simulink model "gimbal_model"  (R2016b)
settings: Solver=VariableStepAuto  StartTime=0.0  StopTime=60  RelTol=1e-3
values from neighbouring files (symbols this model uses):
  A = J*(Omega_phi + Omega)    [IMU.m]
  DIM = data{4}    [gimbal_dynamics.m]
  DIS = data{5}    [gimbal_dynamics.m]
  I1 = data{1}    [gimbal_dynamics.m]    (also in macierze_inercji.m = sym('I1', [4 4]))
  I2 = data{2}    [gimbal_dynamics.m]    (also in macierze_inercji.m = sym('I2', [4 4]))
  I3 = data{3}    [gimbal_dynamics.m]    (also in macierze_inercji.m = sym('I3', [4 4]))
  M = [ud_ucz(3:p-1) ud_ucz(3:p-1).^2 ud_ucz(3:p-1).^3 ud_ucz(2:p-2) ud_ucz(2:p-2).^2 ud_ucz(2:p-2).^3 ud_ucz(1:p-3) ud_ucz(1:p-3).^2 ud_ucz(1:p-3).^3 yd_ucz(3:p-1) yd_ucz(3:p-1).^2 yd_ucz(3:p-1).^3 yd_ucz(2:p-2) yd_ucz(2:p-2).^2 yd_ucz(2:p-2).^3 yd_ucz(1:p-3) yd_ucz(1:p-3).^2 yd_ucz(1:p-3).^3]    [Identification_20191023.m]    (also in MI_beta.m = fillmissing(M,'spline'); gimbal_dynamics.m = data{6}; macierze_inercji.m = sym('M', [1 3]))
  phase = 6    [calculate_PWM.m]    (also in pwm_test.m)
libraries: powerlib x34, simulink x4
settings Model: Creator=Paweł Tymiński  LastModifiedBy=Paweł Tymiński

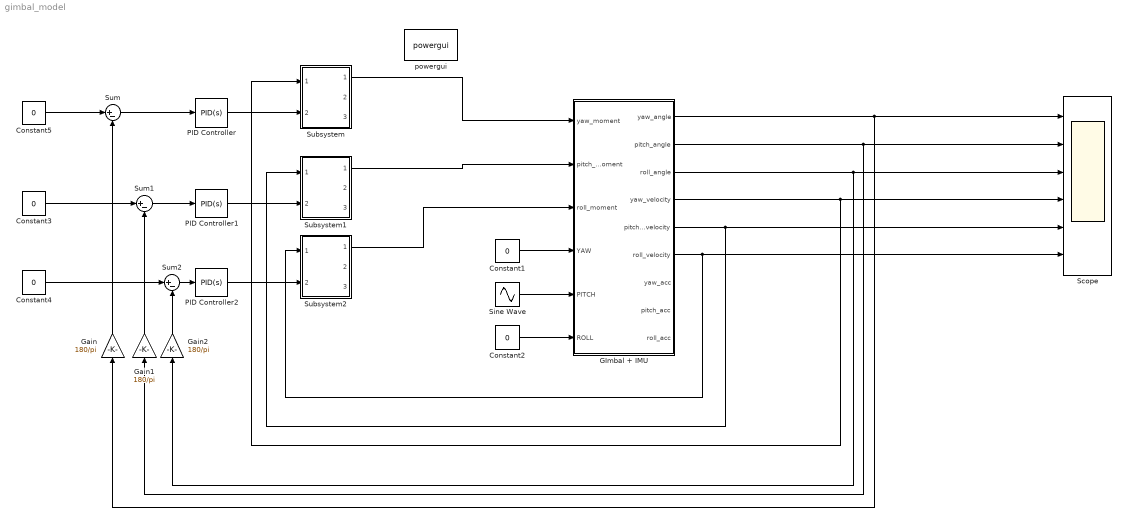
== system gimbal_model ==
  Constant{1..5} (5 alike) : Constant  Value=0
  GImbal + IMU : Subsystem
  Gain : Gain  Gain=180/pi
  Gain1 : Gain  Gain=180/pi
  Gain2 : Gain  Gain=180/pi
  PID Controller : simulink/Continuous/PID Controller  Controller=PID  TimeDomain=Continuous-time  SampleTime=-1  IntegratorMethod=Forward Euler  FilterMethod=Forward Euler  Form=Parallel  UseFilter=on  ControllerParametersSource=internal  P=0.2647  I=1.7647  D=0.0099  N=100  InitialConditionSource=internal  InitialConditionForIntegrator=0  InitialConditionForFilter=0  ExternalReset=none  LimitOutput=off  UpperSaturationLimit=inf  LowerSaturationLimit=-inf  LinearizeAsGain=on  AntiWindupMode=none  Kb=1  TrackingMode=off  Kt=1  PParamMin=[]  PParamMax=[]  IParamMin=[]  IParamMax=[]  DParamMin=[]  DParamMax=[]  NParamMin=[]  NParamMax=[]  KbParamMin=[]  KbParamMax=[]  KtParamMin=[]  KtParamMax=[]  POutMin=[]  POutMax=[]  IOutMin=[]  IOutMax=[]  DOutMin=[]  DOutMax=[]  NOutMin=[]  NOutMax=[]  KbOutMin=[]  KbOutMax=[]  KtOutMin=[]  KtOutMax=[]  IntegratorOutMin=[]  IntegratorOutMax=[]  FilterOutMin=[]  FilterOutMax=[]  SumOutMin=[]  SumOutMax=[]  SumI1OutMin=[]  SumI1OutMax=[]  SumI2OutMin=[]  SumI2OutMax=[]  SumI3OutMin=[]  SumI3OutMax=[]  SumDOutMin=[]  SumDOutMax=[]  SaturationOutMin=[]  SaturationOutMax=[]  IntegratorContinuousStateAttributes=''  IntegratorStateMustResolveToSignalObject=off  IntegratorRTWStateStorageClass=Auto  FilterContinuousStateAttributes=''  FilterStateMustResolveToSignalObject=off  FilterRTWStateStorageClass=Auto  DifferentiatorICPrevScaledInput=0  DifferentiatorOutMin=[]  DifferentiatorOutMax=[]
  PID Controller1 : simulink/Continuous/PID Controller  Controller=PID  TimeDomain=Continuous-time  SampleTime=-1  IntegratorMethod=Forward Euler  FilterMethod=Forward Euler  Form=Parallel  UseFilter=on  ControllerParametersSource=internal  P=0.2353  I=1.5180  D=0.0091  N=100  InitialConditionSource=internal  InitialConditionForIntegrator=0  InitialConditionForFilter=0  ExternalReset=none  LimitOutput=off  UpperSaturationLimit=inf  LowerSaturationLimit=-inf  LinearizeAsGain=on  AntiWindupMode=none  Kb=1  TrackingMode=off  Kt=1  PParamMin=[]  PParamMax=[]  IParamMin=[]  IParamMax=[]  DParamMin=[]  DParamMax=[]  NParamMin=[]  NParamMax=[]  KbParamMin=[]  KbParamMax=[]  KtParamMin=[]  KtParamMax=[]  POutMin=[]  POutMax=[]  IOutMin=[]  IOutMax=[]  DOutMin=[]  DOutMax=[]  NOutMin=[]  NOutMax=[]  KbOutMin=[]  KbOutMax=[]  KtOutMin=[]  KtOutMax=[]  IntegratorOutMin=[]  IntegratorOutMax=[]  FilterOutMin=[]  FilterOutMax=[]  SumOutMin=[]  SumOutMax=[]  SumI1OutMin=[]  SumI1OutMax=[]  SumI2OutMin=[]  SumI2OutMax=[]  SumI3OutMin=[]  SumI3OutMax=[]  SumDOutMin=[]  SumDOutMax=[]  SaturationOutMin=[]  SaturationOutMax=[]  IntegratorContinuousStateAttributes=''  IntegratorStateMustResolveToSignalObject=off  IntegratorRTWStateStorageClass=Auto  FilterContinuousStateAttributes=''  FilterStateMustResolveToSignalObject=off  FilterRTWStateStorageClass=Auto  DifferentiatorICPrevScaledInput=0  DifferentiatorOutMin=[]  DifferentiatorOutMax=[]
  PID Controller2 : simulink/Continuous/PID Controller  Controller=PID  TimeDomain=Continuous-time  SampleTime=-1  IntegratorMethod=Forward Euler  FilterMethod=Forward Euler  Form=Parallel  UseFilter=on  ControllerParametersSource=internal  P=0.2353  I=1.5180  D=0.0091  N=100  InitialConditionSource=internal  InitialConditionForIntegrator=0  InitialConditionForFilter=0  ExternalReset=none  LimitOutput=off  UpperSaturationLimit=inf  LowerSaturationLimit=-inf  LinearizeAsGain=on  AntiWindupMode=none  Kb=1  TrackingMode=off  Kt=1  PParamMin=[]  PParamMax=[]  IParamMin=[]  IParamMax=[]  DParamMin=[]  DParamMax=[]  NParamMin=[]  NParamMax=[]  KbParamMin=[]  KbParamMax=[]  KtParamMin=[]  KtParamMax=[]  POutMin=[]  POutMax=[]  IOutMin=[]  IOutMax=[]  DOutMin=[]  DOutMax=[]  NOutMin=[]  NOutMax=[]  KbOutMin=[]  KbOutMax=[]  KtOutMin=[]  KtOutMax=[]  IntegratorOutMin=[]  IntegratorOutMax=[]  FilterOutMin=[]  FilterOutMax=[]  SumOutMin=[]  SumOutMax=[]  SumI1OutMin=[]  SumI1OutMax=[]  SumI2OutMin=[]  SumI2OutMax=[]  SumI3OutMin=[]  SumI3OutMax=[]  SumDOutMin=[]  SumDOutMax=[]  SaturationOutMin=[]  SaturationOutMax=[]  IntegratorContinuousStateAttributes=''  IntegratorStateMustResolveToSignalObject=off  IntegratorRTWStateStorageClass=Auto  FilterContinuousStateAttributes=''  FilterStateMustResolveToSignalObject=off  FilterRTWStateStorageClass=Auto  DifferentiatorICPrevScaledInput=0  DifferentiatorOutMin=[]  DifferentiatorOutMax=[]
  Scope : Scope  NumInputPorts=6
  Sine Wave : Sin  Amplitude=2  SampleTime=0
  Subsystem : Subsystem
  Subsystem1 : Subsystem
  Subsystem2 : Subsystem
  Sum : Sum  Inputs=|+-
  Sum1 : Sum  Inputs=|+-
  Sum2 : Sum  Inputs=|+-
  powergui : powerlib/powergui  Priority=1  SimulationMode=Discrete  SolverType=Tustin/Backward Euler (TBE)  SampleTime=2e-2  frequency=60  SPID=off  DisableSnubberDevices=off  DisableRonSwitches=off  DisableVfSwitches=off  SwTol=0  DisplayEquations=off  Interpol=off  ExternalGateDelay=off  methode=off  Ts=10  FunctionMessages=off  echomessages=off  HookPort=off  EnableUseOfTLC=off  x0status=blocks  frequencyindice=0  Pbase=100e6  ErrMax=1e-4  Iterations=50  UnitsV=kV  UnitsW=MW  buscounter=0  RestoreLinks=warning  ResistiveCurrentMeasurement=off  Frange=[0:2:500]  Ylog=off  Xlog=on  ShowGrid=off  save=off  variable=ZData  structure=0  ZoomFFT=off  StartTime=0.0  cycles=1  DisplayStyle=1  fundamental=60  FreqAxis=off  MaxFrequency=1000  frequencyindicesteady=1  RmsSteady=1  display=off
  wires:
  Subsystem/1(torque) -> GImbal + IMU/1(yaw_moment)
  Subsystem1/1(torque) -> GImbal + IMU/2(pitch_moment)
  Subsystem2/1(torque) -> GImbal + IMU/3(roll_moment)
  Sum1/1 -> PID Controller1/1
  Sum2/1 -> PID Controller2/1
  Sum/1 -> PID Controller/1
  Gain/1 -> Sum/2
  Gain2/1 -> Sum2/2
  Gain1/1 -> Sum1/2
  Sine Wave/1 -> GImbal + IMU/5(PITCH)
  Constant1/1 -> GImbal + IMU/4(YAW)
  Constant2/1 -> GImbal + IMU/6(ROLL)
  Constant5/1 -> Sum/1
  Constant3/1 -> Sum1/1
  Constant4/1 -> Sum2/1
  GImbal + IMU/4(yaw_velocity) -> Subsystem/1(velocity), Scope/4
  GImbal + IMU/5(pitch_velocity) -> Subsystem1/1(velocity), Scope/5
  GImbal + IMU/6(roll_velocity) -> Subsystem2/1(velocity), Scope/6
  GImbal + IMU/1(yaw_angle) -> Gain/1, Scope/1
  GImbal + IMU/2(pitch_angle) -> Gain1/1, Scope/2
  GImbal + IMU/3(roll_angle) -> Gain2/1, Scope/3
  PID Controller/1 -> Subsystem/2(angle)
  PID Controller1/1 -> Subsystem1/2(angle)
  PID Controller2/1 -> Subsystem2/2(angle)

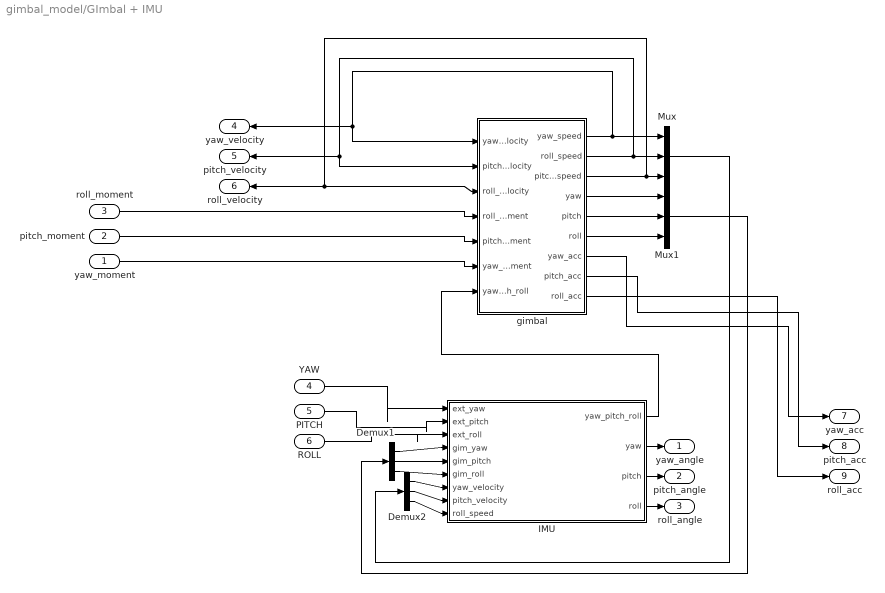
== system gimbal_model/GImbal + IMU ==
  yaw_moment : Inport
  pitch_moment : Inport  Port=2
  roll_moment : Inport  Port=3
  YAW : Inport  Port=4
  PITCH : Inport  Port=5
  ROLL : Inport  Port=6
  Demux1 : Demux  Outputs=3
  Demux2 : Demux  Outputs=3
  IMU : Subsystem
  Mux : Mux  Inputs=3
  Mux1 : Mux  Inputs=3
  gimbal : Subsystem
  yaw_angle : Outport
  pitch_angle : Outport  Port=2
  roll_angle : Outport  Port=3
  yaw_velocity : Outport  Port=4
  pitch_velocity : Outport  Port=5
  roll_velocity : Outport  Port=6
  yaw_acc : Outport  Port=7
  pitch_acc : Outport  Port=8
  roll_acc : Outport  Port=9
  wires:
  gimbal/4(yaw) -> Mux1/1
  gimbal/6(roll) -> Mux1/3
  IMU/3(pitch) -> pitch_angle/1
  YAW/1 -> IMU/1(ext_yaw)
  gimbal/5(pitch) -> Mux1/2
  PITCH/1 -> IMU/2(ext_pitch)
  IMU/2(yaw) -> yaw_angle/1
  IMU/4(roll) -> roll_angle/1
  ROLL/1 -> IMU/3(ext_roll)
  gimbal/2(roll_speed) -> pitch_velocity/1, gimbal/2(pitch_velocity), Mux/2
  gimbal/3(pitch_speed) -> gimbal/3(roll_velocity), roll_velocity/1, Mux/3
  gimbal/1(yaw_speed) -> gimbal/1(yaw_velocity), yaw_velocity/1, Mux/1
  pitch_moment/1 -> gimbal/5(pitch_moment)
  roll_moment/1 -> gimbal/4(roll_moment)
  yaw_moment/1 -> gimbal/6(yaw_moment)
  IMU/1(yaw_pitch_roll) -> gimbal/7(yaw_pitch_roll)
  Demux1/2 -> IMU/5(gim_pitch)
  Demux1/1 -> IMU/4(gim_yaw)
  Demux1/3 -> IMU/6("gim_roll ")
  Demux2/1 -> IMU/7(yaw_velocity)
  Demux2/2 -> IMU/8(pitch_velocity)
  Demux2/3 -> IMU/9(roll_speed)
  Mux1/1 -> Demux1/1
  Mux/1 -> Demux2/1
  gimbal/7(yaw_acc) -> yaw_acc/1
  gimbal/8(pitch_acc) -> pitch_acc/1
  gimbal/9(roll_acc) -> roll_acc/1

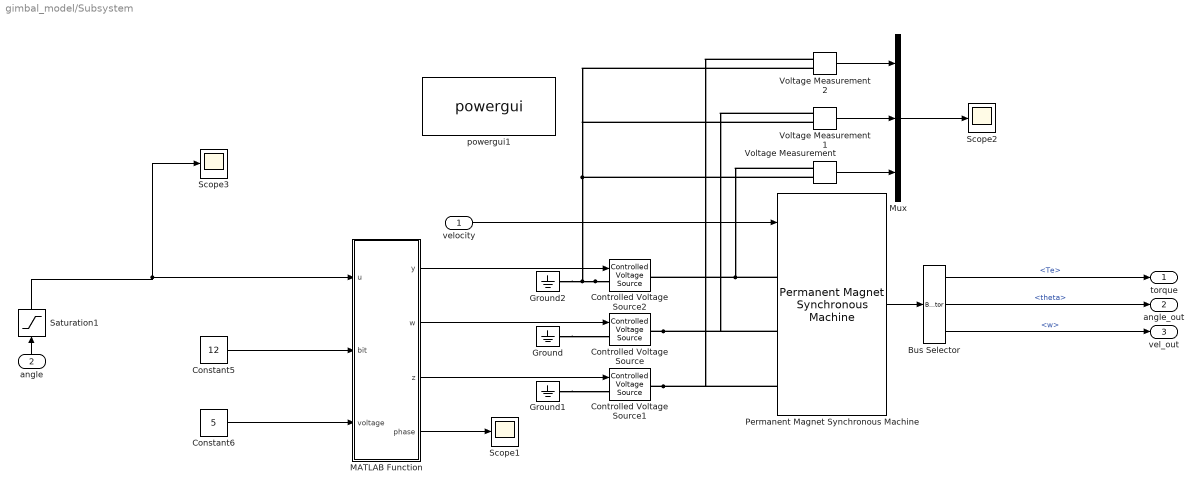
== system gimbal_model/Subsystem ==
  velocity : Inport
  angle : Inport  Port=2
  Bus Selector : BusSelector  OutputSignals=Te,theta,w
  Constant5 : Constant  Value=12
  Constant6 : Constant  Value=5
  Controlled Voltage Source : powerlib/Electrical Sources/Controlled Voltage Source  Initialize=on  Source_Type=DC  Amplitude=12  Phase=0  Frequency=0  Measurements=Voltage
  Controlled Voltage Source1 : powerlib/Electrical Sources/Controlled Voltage Source  Initialize=on  Source_Type=DC  Amplitude=0  Phase=0  Frequency=0  Measurements=None
  Controlled Voltage Source2 : powerlib/Electrical Sources/Controlled Voltage Source  Initialize=on  Source_Type=DC  Amplitude=12  Phase=0  Frequency=0  Measurements=None
  Ground : powerlib/Elements/Ground  LConnTagsString=a
  Ground1 : powerlib/Elements/Ground  LConnTagsString=a
  Ground2 : powerlib/Elements/Ground  LConnTagsString=a
  MATLAB Function : MATLAB Function  TreatAsAtomicUnit=on
  Mux : Mux  Inputs=3
  Permanent Magnet Synchronous Machine : powerlib/Machines/Permanent Magnet Synchronous Machine  NbPhases=3  FluxDistribution=Trapezoidal  RotorType=Round  MechanicalLoad=Speed w  PresetModel=No  ShowDetailedParameters=on  MeasurementBus=on  Resistance=0.023  Inductance=8.5e-3  dqInductances=[8.5e-3,8.5e-3]  La=0.00167  MachineConstant=Flux linkage established by magnets (V.s)  Flux=0.000723497  VoltageCst=1.0607  TorqueCst=0.010129  Flat=120  Mechanical=[0.000621417 4.5 7]  PolePairs=7  InitialConditions=[0,0, 0,0]  InitialConditions5ph=[0 0 0 0 0 0]  TsPowergui=0  TsBlock=0.0003  RefAngle=90 degrees behind phase A axis (modified Park)
  Saturation1 : Saturate  UpperLimit=360
  Scope1 : Scope
  Scope2 : Scope
  Scope3 : Scope
  Voltage Measurement : powerlib/Measurements/Voltage Measurement  PhasorSimulation=off  OutputType=Complex  PSBequivalent=0
  Voltage Measurement1 : powerlib/Measurements/Voltage Measurement  PhasorSimulation=off  OutputType=Complex  PSBequivalent=0
  Voltage Measurement2 : powerlib/Measurements/Voltage Measurement  PhasorSimulation=off  OutputType=Complex  PSBequivalent=0
  powergui1 : powerlib/powergui  Priority=1  SimulationMode=Discrete  SolverType=Tustin/Backward Euler (TBE)  SampleTime=0.0000625  frequency=60  SPID=off  DisableSnubberDevices=off  DisableRonSwitches=off  DisableVfSwitches=off  SwTol=0  DisplayEquations=off  Interpol=off  ExternalGateDelay=off  methode=off  Ts=10  FunctionMessages=off  echomessages=off  HookPort=off  EnableUseOfTLC=off  x0status=blocks  frequencyindice=0  Pbase=100e6  ErrMax=1e-4  Iterations=50  UnitsV=kV  UnitsW=MW  buscounter=0  RestoreLinks=warning  ResistiveCurrentMeasurement=off  Frange=[0:2:500]  Ylog=off  Xlog=on  ShowGrid=off  save=off  variable=ZData  structure=0  ZoomFFT=off  StartTime=0.0  cycles=1  DisplayStyle=1  fundamental=60  FreqAxis=off  MaxFrequency=1000  frequencyindicesteady=1  RmsSteady=1  display=off
  torque : Outport
  angle_out : Outport  Port=2
  vel_out : Outport  Port=3
  wires:
  angle/1 -> Saturation1/1
  velocity/1 -> Permanent Magnet Synchronous Machine/1
  MATLAB Function/1(y) -> Controlled Voltage Source2/1
  Bus Selector/1 -> torque/1  "<Te>"
  Constant6/1 -> MATLAB Function/3(voltage)
  Bus Selector/2 -> angle_out/1  "<theta>"
  MATLAB Function/2(w) -> Controlled Voltage Source/1
  Mux/1 -> Scope2/1
  MATLAB Function/4(phase) -> Scope1/1
  Permanent Magnet Synchronous Machine/1 -> Bus Selector/1
  Voltage Measurement/1 -> Mux/3
  Bus Selector/3 -> vel_out/1  "<w>"
  MATLAB Function/3(z) -> Controlled Voltage Source1/1
  Voltage Measurement2/1 -> Mux/1
  Constant5/1 -> MATLAB Function/2(bit)
  Voltage Measurement1/1 -> Mux/2
  Saturation1/1 -> Scope3/1, MATLAB Function/1(u)
  connections:
  Controlled Voltage Source2/LConn1 -- Ground2/LConn1 -- Voltage Measurement/LConn2 -- Voltage Measurement1/LConn2 -- Voltage Measurement2/LConn2
  Controlled Voltage Source/RConn1 -- Permanent Magnet Synchronous Machine/LConn2 -- Voltage Measurement1/LConn1
  Ground/LConn1 -- Controlled Voltage Source/LConn1
  Ground1/LConn1 -- Controlled Voltage Source1/LConn1
  Voltage Measurement/LConn1 -- Permanent Magnet Synchronous Machine/LConn1 -- Controlled Voltage Source2/RConn1
  Controlled Voltage Source1/RConn1 -- Permanent Magnet Synchronous Machine/LConn3 -- Voltage Measurement2/LConn1

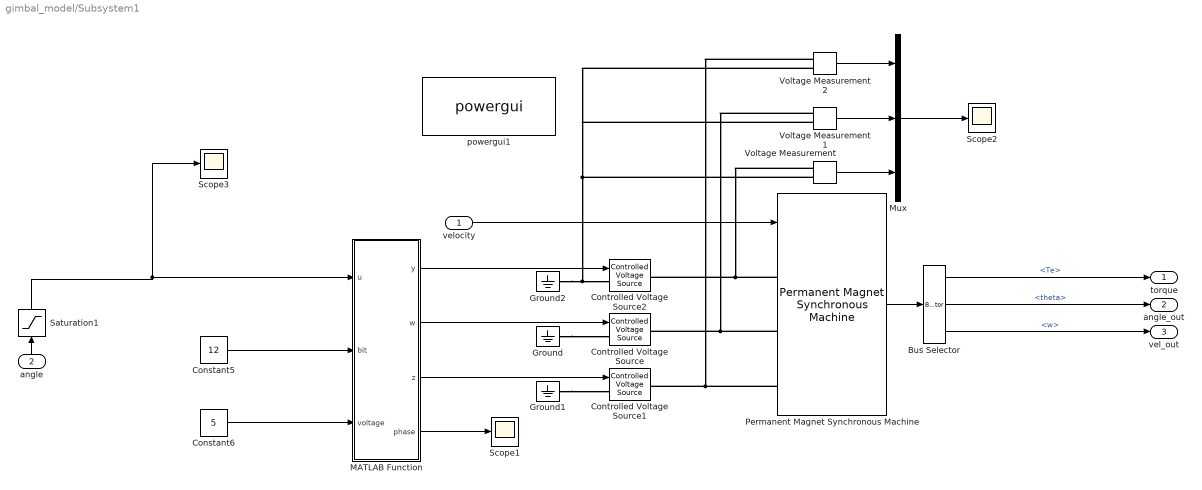
== system gimbal_model/Subsystem1 ==
  velocity : Inport
  angle : Inport  Port=2
  Bus Selector : BusSelector  OutputSignals=Te,theta,w
  Constant5 : Constant  Value=12
  Constant6 : Constant  Value=5
  Controlled Voltage Source : powerlib/Electrical Sources/Controlled Voltage Source  Initialize=on  Source_Type=DC  Amplitude=12  Phase=0  Frequency=0  Measurements=Voltage
  Controlled Voltage Source1 : powerlib/Electrical Sources/Controlled Voltage Source  Initialize=on  Source_Type=DC  Amplitude=0  Phase=0  Frequency=0  Measurements=None
  Controlled Voltage Source2 : powerlib/Electrical Sources/Controlled Voltage Source  Initialize=on  Source_Type=DC  Amplitude=12  Phase=0  Frequency=0  Measurements=None
  Ground : powerlib/Elements/Ground  LConnTagsString=a
  Ground1 : powerlib/Elements/Ground  LConnTagsString=a
  Ground2 : powerlib/Elements/Ground  LConnTagsString=a
  MATLAB Function : MATLAB Function  TreatAsAtomicUnit=on
  Mux : Mux  Inputs=3
  Permanent Magnet Synchronous Machine : powerlib/Machines/Permanent Magnet Synchronous Machine  NbPhases=3  FluxDistribution=Trapezoidal  RotorType=Round  MechanicalLoad=Speed w  PresetModel=No  ShowDetailedParameters=on  MeasurementBus=on  Resistance=0.023  Inductance=8.5e-3  dqInductances=[8.5e-3,8.5e-3]  La=0.00167  MachineConstant=Flux linkage established by magnets (V.s)  Flux=0.000723497  VoltageCst=1.0607  TorqueCst=0.010129  Flat=120  Mechanical=[0.000621417 4.5 7]  PolePairs=7  InitialConditions=[0,0, 0,0]  InitialConditions5ph=[0 0 0 0 0 0]  TsPowergui=0  TsBlock=0.0003  RefAngle=90 degrees behind phase A axis (modified Park)
  Saturation1 : Saturate  UpperLimit=360
  Scope1 : Scope
  Scope2 : Scope
  Scope3 : Scope
  Voltage Measurement : powerlib/Measurements/Voltage Measurement  PhasorSimulation=off  OutputType=Complex  PSBequivalent=0
  Voltage Measurement1 : powerlib/Measurements/Voltage Measurement  PhasorSimulation=off  OutputType=Complex  PSBequivalent=0
  Voltage Measurement2 : powerlib/Measurements/Voltage Measurement  PhasorSimulation=off  OutputType=Complex  PSBequivalent=0
  powergui1 : powerlib/powergui  Priority=1  SimulationMode=Discrete  SolverType=Tustin/Backward Euler (TBE)  SampleTime=0.0000625  frequency=60  SPID=off  DisableSnubberDevices=off  DisableRonSwitches=off  DisableVfSwitches=off  SwTol=0  DisplayEquations=off  Interpol=off  ExternalGateDelay=off  methode=off  Ts=10  FunctionMessages=off  echomessages=off  HookPort=off  EnableUseOfTLC=off  x0status=blocks  frequencyindice=0  Pbase=100e6  ErrMax=1e-4  Iterations=50  UnitsV=kV  UnitsW=MW  buscounter=0  RestoreLinks=warning  ResistiveCurrentMeasurement=off  Frange=[0:2:500]  Ylog=off  Xlog=on  ShowGrid=off  save=off  variable=ZData  structure=0  ZoomFFT=off  StartTime=0.0  cycles=1  DisplayStyle=1  fundamental=60  FreqAxis=off  MaxFrequency=1000  frequencyindicesteady=1  RmsSteady=1  display=off
  torque : Outport
  angle_out : Outport  Port=2
  vel_out : Outport  Port=3
  wires:
  angle/1 -> Saturation1/1
  velocity/1 -> Permanent Magnet Synchronous Machine/1
  MATLAB Function/1(y) -> Controlled Voltage Source2/1
  Bus Selector/1 -> torque/1  "<Te>"
  Constant6/1 -> MATLAB Function/3(voltage)
  Bus Selector/2 -> angle_out/1  "<theta>"
  MATLAB Function/2(w) -> Controlled Voltage Source/1
  Mux/1 -> Scope2/1
  MATLAB Function/4(phase) -> Scope1/1
  Permanent Magnet Synchronous Machine/1 -> Bus Selector/1
  Voltage Measurement/1 -> Mux/3
  Bus Selector/3 -> vel_out/1  "<w>"
  MATLAB Function/3(z) -> Controlled Voltage Source1/1
  Voltage Measurement2/1 -> Mux/1
  Constant5/1 -> MATLAB Function/2(bit)
  Voltage Measurement1/1 -> Mux/2
  Saturation1/1 -> Scope3/1, MATLAB Function/1(u)
  connections:
  Voltage Measurement/LConn2 -- Voltage Measurement1/LConn2 -- Voltage Measurement2/LConn2 -- Controlled Voltage Source2/LConn1 -- Ground2/LConn1
  Voltage Measurement1/LConn1 -- Controlled Voltage Source/RConn1 -- Permanent Magnet Synchronous Machine/LConn2
  Ground/LConn1 -- Controlled Voltage Source/LConn1
  Ground1/LConn1 -- Controlled Voltage Source1/LConn1
  Voltage Measurement/LConn1 -- Controlled Voltage Source2/RConn1 -- Permanent Magnet Synchronous Machine/LConn1
  Voltage Measurement2/LConn1 -- Controlled Voltage Source1/RConn1 -- Permanent Magnet Synchronous Machine/LConn3

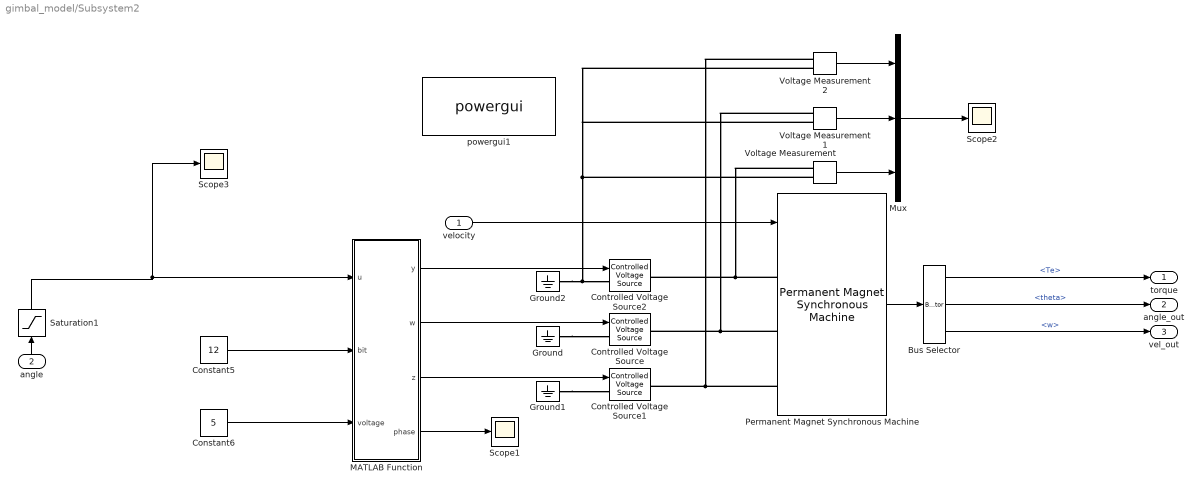
== system gimbal_model/Subsystem2 ==
  velocity : Inport
  angle : Inport  Port=2
  Bus Selector : BusSelector  OutputSignals=Te,theta,w
  Constant5 : Constant  Value=12
  Constant6 : Constant  Value=5
  Controlled Voltage Source : powerlib/Electrical Sources/Controlled Voltage Source  Initialize=on  Source_Type=DC  Amplitude=12  Phase=0  Frequency=0  Measurements=Voltage
  Controlled Voltage Source1 : powerlib/Electrical Sources/Controlled Voltage Source  Initialize=on  Source_Type=DC  Amplitude=0  Phase=0  Frequency=0  Measurements=None
  Controlled Voltage Source2 : powerlib/Electrical Sources/Controlled Voltage Source  Initialize=on  Source_Type=DC  Amplitude=12  Phase=0  Frequency=0  Measurements=None
  Ground : powerlib/Elements/Ground  LConnTagsString=a
  Ground1 : powerlib/Elements/Ground  LConnTagsString=a
  Ground2 : powerlib/Elements/Ground  LConnTagsString=a
  MATLAB Function : MATLAB Function  TreatAsAtomicUnit=on
  Mux : Mux  Inputs=3
  Permanent Magnet Synchronous Machine : powerlib/Machines/Permanent Magnet Synchronous Machine  NbPhases=3  FluxDistribution=Trapezoidal  RotorType=Round  MechanicalLoad=Speed w  PresetModel=No  ShowDetailedParameters=on  MeasurementBus=on  Resistance=0.023  Inductance=8.5e-3  dqInductances=[8.5e-3,8.5e-3]  La=0.00167  MachineConstant=Flux linkage established by magnets (V.s)  Flux=0.000723497  VoltageCst=1.0607  TorqueCst=0.010129  Flat=120  Mechanical=[0.000621417 4.5 7]  PolePairs=7  InitialConditions=[0,0, 0,0]  InitialConditions5ph=[0 0 0 0 0 0]  TsPowergui=0  TsBlock=0.0003  RefAngle=90 degrees behind phase A axis (modified Park)
  Saturation1 : Saturate  UpperLimit=360
  Scope1 : Scope
  Scope2 : Scope
  Scope3 : Scope
  Voltage Measurement : powerlib/Measurements/Voltage Measurement  PhasorSimulation=off  OutputType=Complex  PSBequivalent=0
  Voltage Measurement1 : powerlib/Measurements/Voltage Measurement  PhasorSimulation=off  OutputType=Complex  PSBequivalent=0
  Voltage Measurement2 : powerlib/Measurements/Voltage Measurement  PhasorSimulation=off  OutputType=Complex  PSBequivalent=0
  powergui1 : powerlib/powergui  Priority=1  SimulationMode=Discrete  SolverType=Tustin/Backward Euler (TBE)  SampleTime=0.0000625  frequency=60  SPID=off  DisableSnubberDevices=off  DisableRonSwitches=off  DisableVfSwitches=off  SwTol=0  DisplayEquations=off  Interpol=off  ExternalGateDelay=off  methode=off  Ts=10  FunctionMessages=off  echomessages=off  HookPort=off  EnableUseOfTLC=off  x0status=blocks  frequencyindice=0  Pbase=100e6  ErrMax=1e-4  Iterations=50  UnitsV=kV  UnitsW=MW  buscounter=0  RestoreLinks=warning  ResistiveCurrentMeasurement=off  Frange=[0:2:500]  Ylog=off  Xlog=on  ShowGrid=off  save=off  variable=ZData  structure=0  ZoomFFT=off  StartTime=0.0  cycles=1  DisplayStyle=1  fundamental=60  FreqAxis=off  MaxFrequency=1000  frequencyindicesteady=1  RmsSteady=1  display=off
  torque : Outport
  angle_out : Outport  Port=2
  vel_out : Outport  Port=3
  wires:
  angle/1 -> Saturation1/1
  velocity/1 -> Permanent Magnet Synchronous Machine/1
  MATLAB Function/1(y) -> Controlled Voltage Source2/1
  Bus Selector/1 -> torque/1  "<Te>"
  Constant6/1 -> MATLAB Function/3(voltage)
  Bus Selector/2 -> angle_out/1  "<theta>"
  MATLAB Function/2(w) -> Controlled Voltage Source/1
  Mux/1 -> Scope2/1
  MATLAB Function/4(phase) -> Scope1/1
  Permanent Magnet Synchronous Machine/1 -> Bus Selector/1
  Voltage Measurement/1 -> Mux/3
  Bus Selector/3 -> vel_out/1  "<w>"
  MATLAB Function/3(z) -> Controlled Voltage Source1/1
  Voltage Measurement2/1 -> Mux/1
  Constant5/1 -> MATLAB Function/2(bit)
  Voltage Measurement1/1 -> Mux/2
  Saturation1/1 -> Scope3/1, MATLAB Function/1(u)
  connections:
  Voltage Measurement/LConn2 -- Voltage Measurement1/LConn2 -- Voltage Measurement2/LConn2 -- Controlled Voltage Source2/LConn1 -- Ground2/LConn1
  Voltage Measurement1/LConn1 -- Controlled Voltage Source/RConn1 -- Permanent Magnet Synchronous Machine/LConn2
  Ground/LConn1 -- Controlled Voltage Source/LConn1
  Ground1/LConn1 -- Controlled Voltage Source1/LConn1
  Voltage Measurement/LConn1 -- Controlled Voltage Source2/RConn1 -- Permanent Magnet Synchronous Machine/LConn1
  Voltage Measurement2/LConn1 -- Controlled Voltage Source1/RConn1 -- Permanent Magnet Synchronous Machine/LConn3

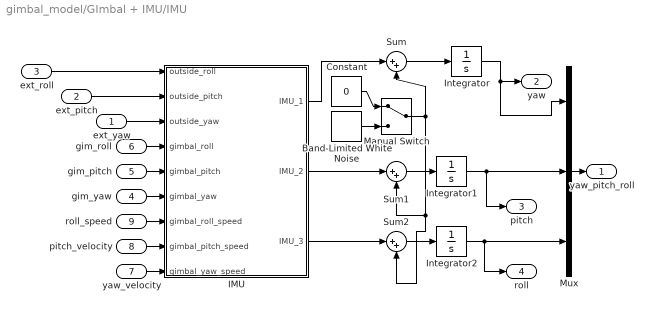
== system gimbal_model/GImbal + IMU/IMU ==
  ext_yaw : Inport
  ext_pitch : Inport  Port=2
  ext_roll : Inport  Port=3
  gim_yaw : Inport  Port=4
  gim_pitch : Inport  Port=5
  "gim_roll " : Inport  Port=6
  yaw_velocity : Inport  Port=7
  pitch_velocity : Inport  Port=8
  roll_speed : Inport  Port=9
  Band-Limited White Noise : simulink/Sources/Band-Limited White Noise  Cov=[0.1]  Ts=0.1  seed=[23341]
  Constant : Constant  Value=0
  IMU : MATLAB Function  TreatAsAtomicUnit=on
  Integrator : Integrator
  Integrator1 : Integrator
  Integrator2 : Integrator
  Manual Switch : ManualSwitch
  Mux : Mux  Inputs=3
  Sum : Sum  Inputs=|++
  Sum1 : Sum  Inputs=|++
  Sum2 : Sum  Inputs=|++
  yaw_pitch_roll : Outport
  yaw : Outport  Port=2
  pitch : Outport  Port=3
  roll : Outport  Port=4
  wires:
  roll_speed/1 -> IMU/7(gimbal_roll_speed)
  gim_pitch/1 -> IMU/5(gimbal_pitch)
  Mux/1 -> yaw_pitch_roll/1
  yaw_velocity/1 -> IMU/9(gimbal_yaw_speed)
  IMU/1(IMU_1) -> Sum/1
  pitch_velocity/1 -> IMU/8(gimbal_pitch_speed)
  ext_pitch/1 -> IMU/2(outside_pitch)
  ext_roll/1 -> IMU/1(outside_roll)
  ext_yaw/1 -> IMU/3(outside_yaw)
  "gim_roll "/1 -> IMU/4(gimbal_roll)
  gim_yaw/1 -> IMU/6(gimbal_yaw)
  IMU/3(IMU_3) -> Sum2/1
  IMU/2(IMU_2) -> Sum1/1
  Integrator2/1 -> roll/1, Mux/3
  Manual Switch/1 -> Sum2/2, Sum1/2, Sum/2
  Sum2/1 -> Integrator2/1
  Sum1/1 -> Integrator1/1
  Sum/1 -> Integrator/1
  Integrator1/1 -> pitch/1, Mux/2
  Integrator/1 -> yaw/1, Mux/1
  Band-Limited White Noise/1 -> Manual Switch/2
  Constant/1 -> Manual Switch/1

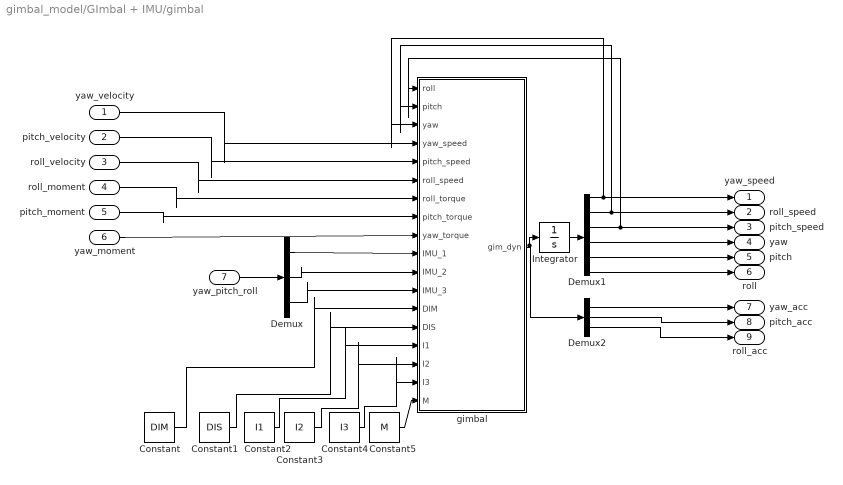
== system gimbal_model/GImbal + IMU/gimbal ==
  yaw_velocity : Inport
  pitch_velocity : Inport  Port=2
  roll_velocity : Inport  Port=3
  roll_moment : Inport  Port=4
  pitch_moment : Inport  Port=5
  yaw_moment : Inport  Port=6
  yaw_pitch_roll : Inport  Port=7
  Constant : Constant  Value=DIM
  Constant1 : Constant  Value=DIS
  Constant2 : Constant  Value=I1
  Constant3 : Constant  Value=I2
  Constant4 : Constant  Value=I3
  Constant5 : Constant  Value=M
  Demux : Demux  Outputs=3
  Demux1 : Demux  Outputs=6
  Demux2 : Demux  Outputs=3
  Integrator : Integrator
  gimbal : MATLAB Function  TreatAsAtomicUnit=on
  yaw_speed : Outport
  roll_speed : Outport  Port=2
  pitch_speed : Outport  Port=3
  yaw : Outport  Port=4
  pitch : Outport  Port=5
  roll : Outport  Port=6
  yaw_acc : Outport  Port=7
  pitch_acc : Outport  Port=8
  roll_acc : Outport  Port=9
  wires:
  Demux/1 -> gimbal/10(IMU_1)
  Demux/3 -> gimbal/12(IMU_3)
  Demux/2 -> gimbal/11(IMU_2)
  gimbal/1(gim_dyn) -> Demux2/1, Integrator/1
  Demux1/2 -> roll_speed/1, gimbal/2(pitch)
  Demux1/1 -> yaw_speed/1, gimbal/3(yaw)
  yaw_pitch_roll/1 -> Demux/1
  pitch_velocity/1 -> gimbal/5(pitch_speed)
  roll_velocity/1 -> gimbal/6(roll_speed)
  roll_moment/1 -> gimbal/7(roll_torque)
  yaw_velocity/1 -> gimbal/4(yaw_speed)
  yaw_moment/1 -> gimbal/9(yaw_torque)
  pitch_moment/1 -> gimbal/8(pitch_torque)
  Demux1/3 -> pitch_speed/1, gimbal/1(roll)
  Integrator/1 -> Demux1/1
  Demux1/6 -> roll/1
  Demux1/5 -> pitch/1
  Demux1/4 -> yaw/1
  Constant5/1 -> gimbal/18(M)
  Constant4/1 -> gimbal/17(I3)
  Constant3/1 -> gimbal/16(I2)
  Constant2/1 -> gimbal/15(I1)
  Constant1/1 -> gimbal/14(DIS)
  Constant/1 -> gimbal/13(DIM)
  Demux2/1 -> yaw_acc/1
  Demux2/2 -> pitch_acc/1
  Demux2/3 -> roll_acc/1

== matlab function gimbal_model/GImbal + IMU/IMU/IMU ==
  data: outside_roll input; IMU_1 output; outside_pitch input; outside_yaw input; gimbal_roll input; gimbal_pitch input; gimbal_yaw input; gimbal_roll_speed input; gimbal_pitch_speed input; gimbal_yaw_speed input; IMU_2 output; IMU_3 output

function [IMU_1, IMU_2, IMU_3] = IMU(outside_roll,outside_pitch,outside_yaw,gimbal_roll , gimbal_pitch , gimbal_yaw , gimbal_roll_speed ,gimbal_pitch_speed , gimbal_yaw_speed )
% kąty gimbala
theta_1 = gimbal_yaw ;
theta_2 = gimbal_pitch ;
theta_3 = gimbal_roll ;

J_0 =[1 0 0;
    0 cos(theta_1) -sin(theta_1);
   -sin(theta_2) cos(theta_2)*sin(theta_1) cos(theta_1)*cos(theta_2)];
Phi_0 = [outside_yaw; outside_pitch; outside_roll];

Omega_phi = J_0*Phi_0;

Omega = [gimbal_yaw_speed; gimbal_pitch_speed; gimbal_roll_speed];

J = [cos(theta_2)*cos(theta_3) sin(theta_3) 0;
    cos(theta_2)*sin(theta_3) cos(theta_3) 0;
    -sin(theta_2) 0 1];
A=J*(Omega_phi + Omega);

IMU_1 = A(1); %yaw
IMU_2 = A(2); %pitch
IMU_3 = A(3); %roll

end

== matlab function gimbal_model/Subsystem/MATLAB Function ==
  data: u input; y output; bit input; voltage input; w output; z output; phase output

function[y,w,z,phase] = calculate_PWM(u,bit,voltage)
%konwersja kąta na wartości sygnału PWM do sterowania silnikiem BLDC
nop = 14;
phase=1;
PWM=0;
resolution = 2^bit; %rozdzielczość bitowa generowanego sygnału
    y=voltage;
    w=voltage;
    z=0;
%kalkulacja wartości PWM na poszczególne fazy

%konwersja kąta na wejściu na radiany
theta_error = deg2rad(u);

%konwersja kąta mechanicznego na elektryczny (poślizg silnika)
theta_e = (theta_error*nop)/2;
%ograniczenie wartości kąta do wartości z zakresu 0-2 pi
theta_e = mod(theta_e,(2*pi));
if(theta_e < 0)
        theta_e = theta_e + (2*pi);
end

  if  theta_e <= 2/6*pi && theta_e>0
    PWM =round(resolution*(tan(theta_e)) /  (sin(2/3*pi)-cos(2/3*pi)*tan(theta_e)));
    phase=1;
elseif theta_e <= 4/6*pi && theta_e>2/6*pi
    PWM =round(resolution*-((tan(theta_e)*cos(2/3*pi)-sin(2/3*pi))/tan(theta_e)));
    phase=2;
elseif theta_e <= 6/6*pi && theta_e>4/6*pi
    PWM =round(resolution*(tan(theta_e)*cos(2/3*pi)-sin(2/3*pi)/sin(4/3*pi) -cos(4/3*pi)*tan(theta_e)));
    phase=3;
elseif theta_e <= 8/6*pi && theta_e>6/6*pi
    PWM =round(resolution*(tan(theta_e)*cos(4/3*pi)-sin(4/3*pi)/sin(2/3*pi) -cos(2/3*pi)*tan(theta_e)));
    phase=4;   
elseif theta_e <= 10/6*pi && theta_e>8/6*pi
    PWM =round(resolution*(sin(4/3*pi) - tan(theta_e)*cos(4/3*pi))/tan(theta_e));
    phase=5;
elseif theta_e <= 12/6*pi && theta_e>10/6*pi
    PWM =round(resolution*(tan(theta_e))/(sin(4/3*pi)-cos(4/3*pi)*tan(theta_e)));
    phase=6;
 end


if(phase==1)
    y=voltage;
    w=(voltage/resolution)*PWM;
    z=0;
elseif(phase==2)
    y=(voltage/resolution)*PWM;
    w=voltage;
    z=0;
elseif(phase==3)
    y=0;
    w=voltage;
    z=(voltage/resolution)*PWM;
elseif(phase==4)
    y=0;
    w=(voltage/resolution)*PWM;
    z=voltage;
elseif(phase==5)
    y=(voltage/resolution)*PWM;
    w=0;
    z=voltage;
else
    y=voltage;
    w=0;
    z=(voltage/resolution)*PWM;
end
end

== matlab function gimbal_model/GImbal + IMU/gimbal/gimbal ==
  data: roll input; gim_dyn output; pitch input; yaw input; yaw_speed input; pitch_speed input; roll_speed input; roll_torque input; pitch_torque input; yaw_torque input; IMU_1 input; IMU_2 input; IMU_3 input; DIM input; DIS input; I1 input; I2 input; I3 input; M input
function gim_dyn = gimbal_dynamics(roll,pitch,yaw,yaw_speed,pitch_speed,roll_speed,roll_torque,pitch_torque,yaw_torque,IMU_1,IMU_2,IMU_3,DIM,DIS,I1,I2,I3,M)

%stała grawitacji
g = 9.81;

%ładowanie macierzy dot. masy i bezwładności gimbala
% data=cell(1,6);
% data = calculate_I_matrix(0);
% I1=data{1};
% I2=data{2};
% I3=data{3};
% DIM=data{4};
% DIS=data{5};
% M=data{6};
%-------------ZMIENNE--------------
% odczyty z IMU
alpha_1 = IMU_1;
alpha_2 = IMU_2;
alpha_3 = IMU_3;
IMU = [alpha_1; alpha_2; alpha_3];

% momenty generowane przez silnik - zmienne sterujace
 T1 = yaw_torque ;
 T2 = pitch_torque ;
 T3 = roll_torque ;
%predkosci katowe osiagane przez gimbal
 om_1 = yaw_speed ;
 om_2 = pitch_speed ;
 om_3 = roll_speed ;
Omega = [om_1; om_2; om_3];
%kąty osiagane aktualnie przez gimbal
 theta_1 = yaw ;
 theta_2 = pitch ;
 theta_3 = roll ;
    THETA = [theta_1; theta_2; theta_3];

%---------------FUNKCJE---------------------

H = calculate_H_matrix(THETA,Omega,I1,I2,I3,DIM);
D = calculate_D_matrix(THETA,I1,I2,I3,DIM);
Q = calculate_Q_matrix(T1,T2,T3,Omega);
G = calculate_G_matrix(IMU,THETA,DIM,g,M,DIS);

gim_dyn = [inv(D)\(Q-H-G); Omega];
end

== matlab function gimbal_model/Subsystem1/MATLAB Function ==
  data: u input; y output; bit input; voltage input; w output; z output; phase output

function[y,w,z,phase] = calculate_PWM(u,bit,voltage)
%konwersja kąta na wartości sygnału PWM do sterowania silnikiem BLDC
nop = 14;
phase=1;
PWM=0;
resolution = 2^bit; %rozdzielczość bitowa generowanego sygnału
    y=voltage;
    w=voltage;
    z=0;
%kalkulacja wartości PWM na poszczególne fazy

%konwersja kąta na wejściu na radiany
theta_error = deg2rad(u);

%konwersja kąta mechanicznego na elektryczny (poślizg silnika)
theta_e = (theta_error*nop)/2;
%ograniczenie wartości kąta do wartości z zakresu 0-2 pi
theta_e = mod(theta_e,(2*pi));
if(theta_e < 0)
        theta_e = theta_e + (2*pi);
end

  if  theta_e <= 2/6*pi && theta_e>0
    PWM =round(resolution*(tan(theta_e)) /  (sin(2/3*pi)-cos(2/3*pi)*tan(theta_e)));
    phase=1;
elseif theta_e <= 4/6*pi && theta_e>2/6*pi
    PWM =round(resolution*-((tan(theta_e)*cos(2/3*pi)-sin(2/3*pi))/tan(theta_e)));
    phase=2;
elseif theta_e <= 6/6*pi && theta_e>4/6*pi
    PWM =round(resolution*(tan(theta_e)*cos(2/3*pi)-sin(2/3*pi)/sin(4/3*pi) -cos(4/3*pi)*tan(theta_e)));
    phase=3;
elseif theta_e <= 8/6*pi && theta_e>6/6*pi
    PWM =round(resolution*(tan(theta_e)*cos(4/3*pi)-sin(4/3*pi)/sin(2/3*pi) -cos(2/3*pi)*tan(theta_e)));
    phase=4;   
elseif theta_e <= 10/6*pi && theta_e>8/6*pi
    PWM =round(resolution*(sin(4/3*pi) - tan(theta_e)*cos(4/3*pi))/tan(theta_e));
    phase=5;
elseif theta_e <= 12/6*pi && theta_e>10/6*pi
    PWM =round(resolution*(tan(theta_e))/(sin(4/3*pi)-cos(4/3*pi)*tan(theta_e)));
    phase=6;
 end


if(phase==1)
    y=voltage;
    w=(voltage/resolution)*PWM;
    z=0;
elseif(phase==2)
    y=(voltage/resolution)*PWM;
    w=voltage;
    z=0;
elseif(phase==3)
    y=0;
    w=voltage;
    z=(voltage/resolution)*PWM;
elseif(phase==4)
    y=0;
    w=(voltage/resolution)*PWM;
    z=voltage;
elseif(phase==5)
    y=(voltage/resolution)*PWM;
    w=0;
    z=voltage;
else
    y=voltage;
    w=0;
    z=(voltage/resolution)*PWM;
end
end

== matlab function gimbal_model/Subsystem2/MATLAB Function ==
  data: u input; y output; bit input; voltage input; w output; z output; phase output

function[y,w,z,phase] = calculate_PWM(u,bit,voltage)
%konwersja kąta na wartości sygnału PWM do sterowania silnikiem BLDC
nop = 14;
phase=1;
PWM=0;
resolution = 2^bit; %rozdzielczość bitowa generowanego sygnału
    y=voltage;
    w=voltage;
    z=0;
%kalkulacja wartości PWM na poszczególne fazy

%konwersja kąta na wejściu na radiany
theta_error = deg2rad(u);

%konwersja kąta mechanicznego na elektryczny (poślizg silnika)
theta_e = (theta_error*nop)/2;
%ograniczenie wartości kąta do wartości z zakresu 0-2 pi
theta_e = mod(theta_e,(2*pi));
if(theta_e < 0)
        theta_e = theta_e + (2*pi);
end

  if  theta_e <= 2/6*pi && theta_e>0
    PWM =round(resolution*(tan(theta_e)) /  (sin(2/3*pi)-cos(2/3*pi)*tan(theta_e)));
    phase=1;
elseif theta_e <= 4/6*pi && theta_e>2/6*pi
    PWM =round(resolution*-((tan(theta_e)*cos(2/3*pi)-sin(2/3*pi))/tan(theta_e)));
    phase=2;
elseif theta_e <= 6/6*pi && theta_e>4/6*pi
    PWM =round(resolution*(tan(theta_e)*cos(2/3*pi)-sin(2/3*pi)/sin(4/3*pi) -cos(4/3*pi)*tan(theta_e)));
    phase=3;
elseif theta_e <= 8/6*pi && theta_e>6/6*pi
    PWM =round(resolution*(tan(theta_e)*cos(4/3*pi)-sin(4/3*pi)/sin(2/3*pi) -cos(2/3*pi)*tan(theta_e)));
    phase=4;   
elseif theta_e <= 10/6*pi && theta_e>8/6*pi
    PWM =round(resolution*(sin(4/3*pi) - tan(theta_e)*cos(4/3*pi))/tan(theta_e));
    phase=5;
elseif theta_e <= 12/6*pi && theta_e>10/6*pi
    PWM =round(resolution*(tan(theta_e))/(sin(4/3*pi)-cos(4/3*pi)*tan(theta_e)));
    phase=6;
 end


if(phase==1)
    y=voltage;
    w=(voltage/resolution)*PWM;
    z=0;
elseif(phase==2)
    y=(voltage/resolution)*PWM;
    w=voltage;
    z=0;
elseif(phase==3)
    y=0;
    w=voltage;
    z=(voltage/resolution)*PWM;
elseif(phase==4)
    y=0;
    w=(voltage/resolution)*PWM;
    z=voltage;
elseif(phase==5)
    y=(voltage/resolution)*PWM;
    w=0;
    z=voltage;
else
    y=voltage;
    w=0;
    z=(voltage/resolution)*PWM;
end
end
